simulink model "test_memristor_vteam_v2_linear"  (R2018a)
settings: Solver=VariableStepAuto  StartTime=0.0  StopTime=2  FixedStep=1e-4  MaxStep=1e-4  MinStep=1e-9  RelTol=1e-3  AbsTol=1e-6
libraries: fl_lib x4, nesl_utility x3, simulink x1
settings Model: Creator=bici  LastModifiedBy=bici
settings SolverCC: InitialStep=1e-9
settings DataIOCC: SaveState=on  InspectSignalLogs=on
settings SimscapeCC: SimscapeNormalizeSystem=off

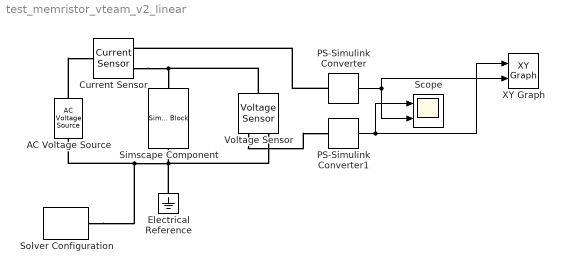
== system test_memristor_vteam_v2_linear ==
  AC Voltage Source : fl_lib/Electrical/Electrical Sources/AC Voltage Source  amp=6 V  shift=0 deg  frequency=0.5 Hz  omega=0 rad/s
  Current Sensor : fl_lib/Electrical/Electrical Sensors/Current Sensor
  Electrical Reference : fl_lib/Electrical/Electrical Elements/Electrical Reference
  PS-Simulink Converter : nesl_utility/PS-Simulink Converter  PhysicalDomain=network_engine_domain  SubClassName=ps_output  LeftPortType=input  RightPortType=output  PseudoPeriodic=off  Frequencies=[]  Unit=1  AffineConversion=off
  PS-Simulink Converter1 : nesl_utility/PS-Simulink Converter  PhysicalDomain=network_engine_domain  SubClassName=ps_output  LeftPortType=input  RightPortType=output  PseudoPeriodic=off  Frequencies=[]  Unit=1  AffineConversion=off
  Scope : Scope  NumInputPorts=2
  Simscape Component : SimscapeComponentBlock  SourceFile=memristor_vteam_v2_linear  ComponentPath=memristor_vteam_v2_linear  ComponentVariants=memristor_vteam_v2_linear  ComponentVariantNames=memristor_vteam_v2_linear  ClassName=memristor_vteam_v2_linear  SchemaVersion=1  k_off=1e-4 m/s  v_off=1.4 V  a_off=5  k_on=-30 m/s  v_on=-5.7 V  a_on=5  R_off=5e7 Ohm  w_off=10e-9 m  R_on=1.5e5 Ohm  w_on=0 m  i_specify=off  i_priority=None  i=0 A  i_nominal_specify=off  i_nominal_unit=A  i_nominal_value=1  v_specify=off  v_priority=None  v=0 V  v_nominal_specify=off  v_nominal_unit=V  v_nominal_value=1  dwoff_p_specify=off  dwoff_p_priority=None  dwoff_p=0 m/s  dwoff_p_nominal_specify=off  dwoff_p_nominal_unit=m/s  dwoff_p_nominal_value=1  dwonn_p_specify=off  dwonn_p_priority=None  dwonn_p=0 m/s  dwonn_p_nominal_specify=off  dwonn_p_nominal_unit=m/s  dwonn_p_nominal_value=1
      settings: CopyFcn=simscape.engine.sli.internal.componentblockcallback(gcbh,'COPY')  PreCopyFcn=simscape.engine.sli.internal.componentblockcallback(gcbh,'PRECOPY')  PreDeleteFcn=simscape.engine.sli.internal.componentblockcallback(gcbh,'PREDELETE')
      mask Type: memristor_vteam_v2_linear
      mask Display:
      | disp('Simscape\n\n\n')
      | disp('\n\n\nmemristor_vteam_v2_linear');
      | color('red');
      | port_label('RConn', 1,'-');
      | port_label('LConn', 1,'+');
  Solver Configuration : nesl_utility/Solver Configuration  PhysicalDomain=network_engine_domain  SubClassName=solver  LeftPortType=input  RightPortType=generic  Tones=[]  Harmonics=[]  SimulateNoise=off  Profile=off  UseLocalSampling=off  EnableSwitchedLinearOptims=on  FrequencyDomain=off  UseCCode=off  RelTol=0.001  AbsTol=1e-06  MinStep=1e-09  ToWorkspace=off  RevertToSquareIcSolve=off  NumHomotopyIterations=100  PhasorMode=off  PhasorModeNumHarmonics=1  DoDC=off  ResidualTolerance=1e-09  UseLocalSolver=off  LocalSolverChoice=NE_BACKWARD_EULER_ADVANCER  LocalSolverSampleTime=0.001  DoFixedCost=off  MaxNonlinIter=3  MaxModeIter=2  LinearAlgebra=Sparse  EquationFormulation=NE_TIME_EF  DelaysMemoryBudget=1024  AutomaticFiltering=on  FilteringTimeConstant=0.001
  Voltage Sensor : fl_lib/Electrical/Electrical Sensors/Voltage Sensor
  XY Graph : simulink/Sinks/XY Graph  xmin=-8  xmax=6  ymin=-0.00005  ymax=0.00002  st=-1
  wires:
  PS-Simulink Converter/1 -> Scope/2, XY Graph/2
  PS-Simulink Converter1/1 -> Scope/1, XY Graph/1
  connections:
  Solver Configuration/RConn1 -- AC Voltage Source/RConn1 -- Voltage Sensor/RConn2 -- Simscape Component/RConn1 -- Electrical Reference/LConn1
  Current Sensor/RConn2 -- Voltage Sensor/LConn1 -- Simscape Component/LConn1
  PS-Simulink Converter/LConn1 -- Current Sensor/RConn1
  Voltage Sensor/RConn1 -- PS-Simulink Converter1/LConn1
  AC Voltage Source/LConn1 -- Current Sensor/LConn1
